simulink model "verify_Pressure_Drop_Collector_mdl"  (R2016b)
settings: Solver=FixedStepDiscrete  StartTime=0.0  StopTime=3  FixedStep=1  MaxStep=1  RelTol=1e-3  EnableMultiTasking=on
libraries: carnot x3, simulink x1
settings Model: Creator=drhf  LastModifiedBy=drhf
settings DataIOCC: LimitDataPoints=on  SaveFormat=Array  SignalLoggingSaveFormat=ModelDataLogs
settings OptimizationCC: ExpressionDepthLimit=2147483647  LifeSpan=inf
settings DebuggingCC: UnderspecifiedInitializationDetection=Classic  MergeDetectMultiDrivingBlocksExec=none  SolverPrmCheckMsg=warning  FcnCallInpInsideContextMsg=warning  StateNameClashWarn=warning  SFUnexpectedBacktrackingDiag=warning  SFNoUnconditionalDefaultTransitionDiag=warning  SFExecutionAtInitializationDiag=none
settings HardwareCC: ProdBitPerPointer=32  ProdBitPerSizeT=32  ProdBitPerPtrDiffT=32  ProdLargestAtomicFloat=None  ProdIntDivRoundTo=Undefined  ProdEndianess=Unspecified  ProdWordSize=32  ProdHWDeviceType=32-bit Generic
settings ModelReferenceCC: PropagateSignalLabelsOutOfModel=off
settings GRTTargetCC: TargetLangStandard=C89/C90 (ANSI)  GeneratePreprocessorConditionals=Disable all  CombineOutputUpdateFcns=off  GRTInterface=on
settings ConfigComp: CovMetricSettings=dw  CovHtmlReporting=on  CovSaveCumulativeToWorkspaceVar=on  CovSaveSingleToWorkspaceVar=on  CovExternalEMLEnable=off

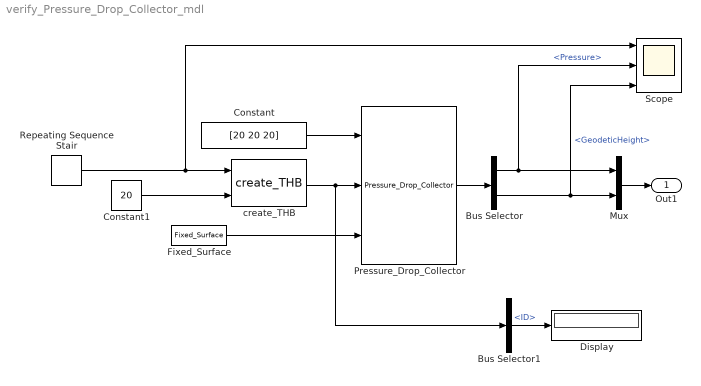
== system verify_Pressure_Drop_Collector_mdl ==
  Bus Selector : BusSelector  OutputSignals=Pressure,GeodeticHeight
  Bus Selector1 : BusSelector  OutputSignals=ID
  Constant : Constant  Value=[20 20 20]
  Constant1 : Constant  Value=20
  Display : Display
  Fixed_Surface : carnot/Weather/Fixed_Surface  colangle=30  colazi=0  colrot=0
  Mux : Mux  Inputs=2
  Pressure_Drop_Collector : carnot/Basic/Pressure_Drop/Pressure_Drop_Collector  len=1  lin=10  qua=10
  Repeating Sequence Stair : simulink/Sources/Repeating Sequence Stair  OutValues=[0 300 900]/3600  tsamp=-1  OutMin=[]  OutMax=[]  OutDataTypeStr=double  OutputDataTypeScalingMode=double  OutDataType=fixdt(0,8)  ConRadixGroup=Best Precision: Vector-wise  OutScaling=2^-12
  Scope : Scope  NumInputPorts=3
  create_THB : carnot/Source/Simple/create_THB  p=2e5  fluid=Water  mix=0  mix2=0  mix3=0  dia=0.02  hgt=0  mID=Full Pressure Drop with Static Height
  Out1 : Outport
  wires:
  create_THB/1 -> Bus Selector1/1, Pressure_Drop_Collector/2
  Pressure_Drop_Collector/1 -> Bus Selector/1
  Bus Selector/1 -> Scope/2, Mux/1  "<Pressure>"
  Constant/1 -> Pressure_Drop_Collector/1
  Fixed_Surface/1 -> Pressure_Drop_Collector/3
  Repeating Sequence Stair/1 -> Scope/1, create_THB/1
  Constant1/1 -> create_THB/2
  Mux/1 -> Out1/1
  Bus Selector/2 -> Scope/3, Mux/2  "<GeodeticHeight>"
  Bus Selector1/1 -> Display/1  "<ID>"
